simulink model "vehicle_model"  (R2020b)
settings: Solver=VariableStepAuto  StartTime=0.0  StopTime=10.0  RelTol=1e-3
model workspace (MAT data in the model file):
  Gravity = 0
  Mass = 0
  Steering_ratio = 0
  Track_width_front = 0
  Track_width_rear = 0
  Weight_dist_front = 0
  Wheelbase = 0
libraries: simulink_extras x3
settings Model: OrderedModelArguments=off  Creator=Matthew  LastModifiedBy=User

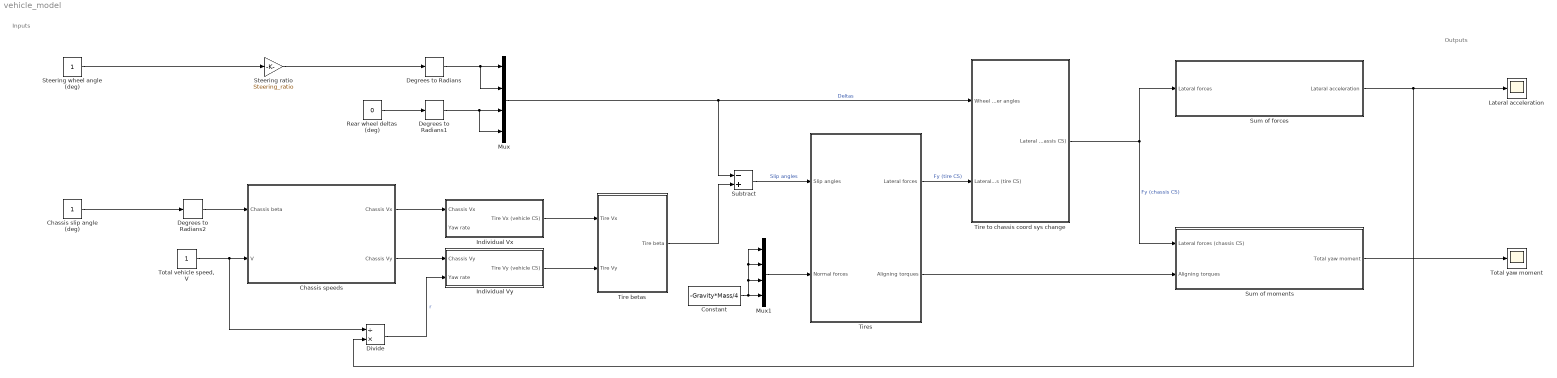
== system vehicle_model ==
  note: Outputs
  note: Inputs
  Chassis slip angle (deg) : Constant
  Chassis speeds : Subsystem
  Constant : Constant  Value=-Gravity*Mass/4
  Degrees to Radians : simulink_extras/Transformations/Degrees to Radians
  Degrees to Radians1 : simulink_extras/Transformations/Degrees to Radians
  Degrees to Radians2 : simulink_extras/Transformations/Degrees to Radians
  Divide : Product  Inputs=/*
  "Individual Vx " : Subsystem
  Individual Vy : Subsystem
  Lateral acceleration : Scope
  Mux : Mux
  Mux1 : Mux
  Rear wheel deltas (deg) : Constant  Value=0
  Steering ratio : Gain  Gain=Steering_ratio
  Steering wheel angle (deg) : Constant
  Subtract : Sum  Inputs=-+
  Sum of forces : Subsystem
  Sum of moments : Subsystem
  Tire betas : Subsystem
  Tire to chassis coord sys change : Subsystem
  Tires : Subsystem
  "Total vehicle speed, V" : Constant
  Total yaw moment : Scope
  wires:
  Tires/1(Lateral forces) -> Tire to chassis coord sys change/2(Lateral forces (tire CS))  "Fy (tire CS)"
  Mux/1 -> Tire to chassis coord sys change/1(Wheel steer angles), Subtract/1  "Deltas"
  Steering ratio/1 -> Degrees to Radians/1
  Degrees to Radians/1 -> Mux/1, Mux/2
  Rear wheel deltas (deg)/1 -> Degrees to Radians1/1
  Degrees to Radians1/1 -> Mux/3, Mux/4
  Chassis speeds/1(Chassis Vx) -> "Individual Vx "/1(Chassis Vx)
  Chassis speeds/2(Chassis Vy) -> Individual Vy/1(Chassis Vy)
  "Individual Vx "/1(Tire Vx (vehicle CS)) -> Tire betas/1(Tire Vx)
  Individual Vy/1(Tire Vy (vehicle CS)) -> Tire betas/2(Tire Vy)
  Tire betas/1(Tire beta) -> Subtract/2
  Subtract/1 -> Tires/1(Slip angles)  "Slip angles"
  Steering wheel angle (deg)/1 -> Steering ratio/1
  Degrees to Radians2/1 -> Chassis speeds/1(Chassis beta)
  Chassis slip angle (deg)/1 -> Degrees to Radians2/1
  "Total vehicle speed, V"/1 -> Divide/1, Chassis speeds/2(V)
  Tire to chassis coord sys change/1(Lateral forces (chassis CS)) -> Sum of moments/1(Lateral forces (chassis CS)), Sum of forces/1(Lateral forces)  "Fy (chassis CS)"
  Tires/2(Aligning torques) -> Sum of moments/2(Aligning torques)
  Sum of forces/1(Lateral acceleration) -> Divide/2, Lateral acceleration/1
  Sum of moments/1(Total yaw moment) -> Total yaw moment/1
  Divide/1 -> Individual Vy/2(Yaw rate)  "r"
  Mux1/1 -> Tires/2(Normal forces)
  Constant/1 -> Mux1/1, Mux1/2, Mux1/3, Mux1/4

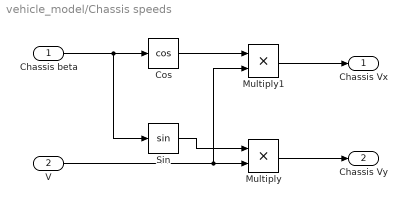
== system vehicle_model/Chassis speeds ==
  Chassis beta : Inport
  V : Inport  Port=2
  Cos : Trigonometry  Operator=cos
  Multiply : Product  Inputs=**
  Multiply1 : Product  Inputs=**
  Sin : Trigonometry
  Chassis Vx : Outport
  Chassis Vy : Outport  Port=2
  wires:
  Multiply/1 -> Chassis Vy/1
  Chassis beta/1 -> Sin/1, Cos/1
  V/1 -> Multiply1/2, Multiply/2
  Sin/1 -> Multiply/1
  Cos/1 -> Multiply1/1
  Multiply1/1 -> Chassis Vx/1

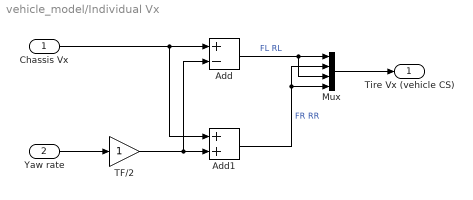
== system vehicle_model/Individual Vx  ==
  Chassis Vx : Inport
  Yaw rate : Inport  Port=2
  Add : Sum  Inputs=+-
  Add1 : Sum
  Mux : Mux
  TF/2 : Gain
  Tire Vx (vehicle CS) : Outport
  wires:
  Chassis Vx/1 -> Add1/1, Add/1
  Yaw rate/1 -> TF/2/1
  TF/2/1 -> Add/2, Add1/2
  Add/1 -> Mux/3, Mux/1  "FL RL"
  Add1/1 -> Mux/4, Mux/2  "FR RR"
  Mux/1 -> Tire Vx (vehicle CS)/1

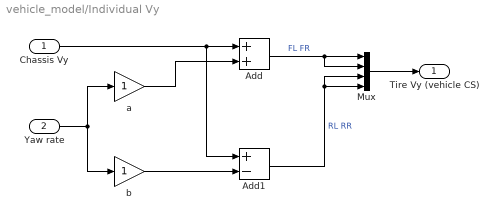
== system vehicle_model/Individual Vy ==
  Chassis Vy : Inport
  Yaw rate : Inport  Port=2
  Add : Sum
  Add1 : Sum  Inputs=+-
  Mux : Mux
  a : Gain
  b : Gain
  Tire Vy (vehicle CS) : Outport
  wires:
  Chassis Vy/1 -> Add1/1, Add/1
  Yaw rate/1 -> b/1, a/1
  a/1 -> Add/2
  Mux/1 -> Tire Vy (vehicle CS)/1
  Add/1 -> Mux/2, Mux/1  "FL FR"
  b/1 -> Add1/2
  Add1/1 -> Mux/4, Mux/3  "RL RR"

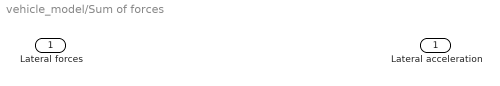
== system vehicle_model/Sum of forces ==
  Lateral forces : Inport
  Lateral acceleration : Outport

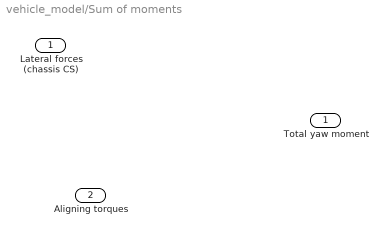
== system vehicle_model/Sum of moments ==
  Lateral forces (chassis CS) : Inport
  Aligning torques : Inport  Port=2
  Total yaw moment : Outport

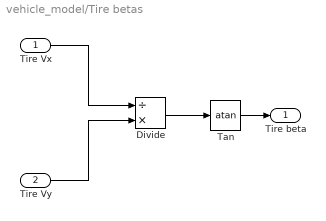
== system vehicle_model/Tire betas ==
  Tire Vx : Inport
  Tire Vy : Inport  Port=2
  Divide : Product  Inputs=/*
  Tan : Trigonometry  Operator=atan
  Tire beta : Outport
  wires:
  Tire Vy/1 -> Divide/2
  Tire Vx/1 -> Divide/1
  Divide/1 -> Tan/1
  Tan/1 -> Tire beta/1

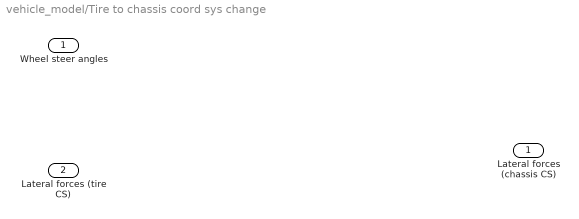
== system vehicle_model/Tire to chassis coord sys change ==
  Wheel steer angles : Inport
  Lateral forces (tire CS) : Inport  Port=2
  Lateral forces (chassis CS) : Outport

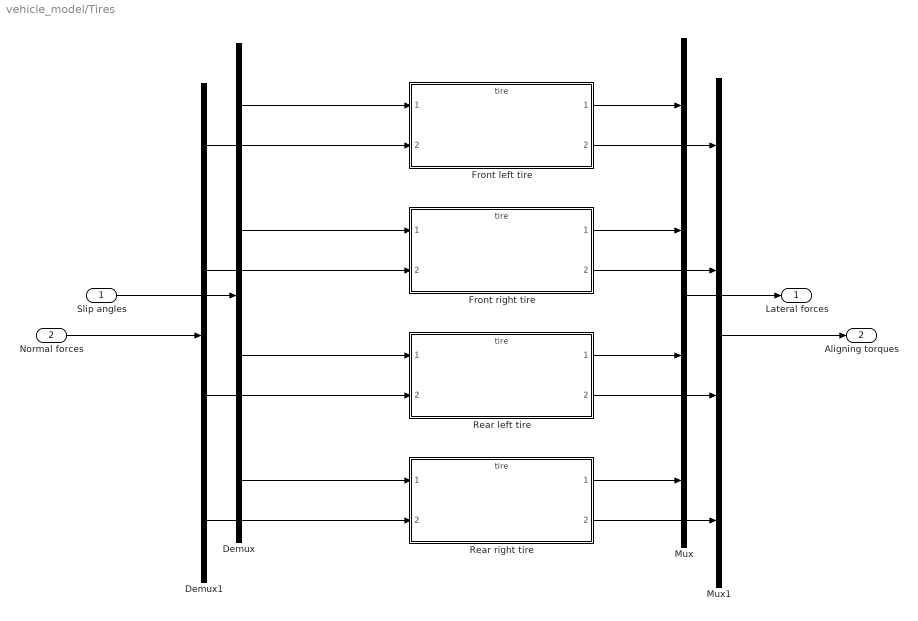
== system vehicle_model/Tires ==
  Slip angles : Inport
  Normal forces : Inport  Port=2
  Demux : Demux
  Demux1 : Demux
  Front left tire : ModelReference  ModelNameDialog=tire.slx  SimulationMode=Normal  ModelReferenceVersion=1.1
  Front right tire : ModelReference  ModelNameDialog=tire.slx  SimulationMode=Normal  ModelReferenceVersion=1.1
  Mux : Mux
  Mux1 : Mux
  Rear left tire : ModelReference  ModelNameDialog=tire.slx  SimulationMode=Normal  ModelReferenceVersion=1.1
  Rear right tire : ModelReference  ModelNameDialog=tire.slx  SimulationMode=Normal  ModelReferenceVersion=1.1
  Lateral forces : Outport
  Aligning torques : Outport  Port=2
  wires:
  Slip angles/1 -> Demux/1
  Demux/1 -> Front left tire/1
  Demux/2 -> Front right tire/1
  Demux/3 -> Rear left tire/1
  Demux/4 -> Rear right tire/1
  Demux1/1 -> Front left tire/2
  Demux1/2 -> Front right tire/2
  Demux1/3 -> Rear left tire/2
  Demux1/4 -> Rear right tire/2
  Normal forces/1 -> Demux1/1
  Mux/1 -> Lateral forces/1
  Front left tire/1 -> Mux/1
  Front right tire/1 -> Mux/2
  Rear left tire/1 -> Mux/3
  Rear right tire/1 -> Mux/4
  Front left tire/2 -> Mux1/1
  Front right tire/2 -> Mux1/2
  Rear left tire/2 -> Mux1/3
  Rear right tire/2 -> Mux1/4
  Mux1/1 -> Aligning torques/1
